simulink model "case3"  (R2024b)
settings: Solver=FixedStepAuto  StartTime=0  StopTime=1  FixedStep=1e-7  RelTol=1e-3
values from neighbouring files (symbols this model uses):
  SG_D_1_D = 0.01056    [IEEE9_case_parameters.m]    (also in case1_parameters.m; case2_parameters.m; case3_parameters.m; case4_parameters.m)
  SG_D_1_EnableSaturation = 0    [IEEE9_case_parameters.m]    (also in case1_parameters.m; case2_parameters.m; case3_parameters.m; case4_parameters.m)
  SG_D_1_f0 = 60    [IEEE9_case_parameters.m]    (also in case1_parameters.m; case2_parameters.m; case3_parameters.m; case4_parameters.m)
  SG_D_1_H = 7.5    [IEEE9_case_parameters.m]    (also in case1_parameters.m; case2_parameters.m; case3_parameters.m; case4_parameters.m)
  SG_D_1_K_A = 20    [IEEE9_case_parameters.m]    (also in case1_parameters.m; case2_parameters.m; case3_parameters.m; case4_parameters.m)
  SG_D_1_K_E = 1.000000e+1    (= 10)    [IEEE9_case_parameters.m]    (also in case1_parameters.m; case2_parameters.m; case3_parameters.m; case4_parameters.m)
  SG_D_1_K_F = 2.363    [IEEE9_case_parameters.m]    (also in case1_parameters.m; case2_parameters.m; case3_parameters.m; case4_parameters.m)
  SG_D_1_K_s = 0.5    [IEEE9_case_parameters.m]    (also in case1_parameters.m = 5; case2_parameters.m = 5; case3_parameters.m = 5; case4_parameters.m = 5)
  SG_D_1_R_a = 0.001088    [IEEE9_case_parameters.m]    (also in case1_parameters.m; case2_parameters.m; case3_parameters.m; case4_parameters.m)
  SG_D_1_S_A = 1    [IEEE9_case_parameters.m]    (also in case1_parameters.m; case2_parameters.m; case3_parameters.m; case4_parameters.m)
  SG_D_1_S_B = 0.103    [IEEE9_case_parameters.m]    (also in case1_parameters.m; case2_parameters.m; case3_parameters.m; case4_parameters.m)
  SG_D_1_S_N = 10.659857    [IEEE9_case_parameters.m]    (also in case1_parameters.m; case2_parameters.m; case3_parameters.m; case4_parameters.m)
  SG_D_1_SpeedPara = 200    [IEEE9_case_parameters.m]    (also in case1_parameters.m; case2_parameters.m; case3_parameters.m; case4_parameters.m)
  SG_D_1_T_0 = 0.720173    [IEEE9_case_parameters.m]    (also in case1_parameters.m = 0.755522; case2_parameters.m = 0.808931; case3_parameters.m = 0.869402; case4_parameters.m = 0.729316)
  SG_D_1_T_1 = 0.3    [IEEE9_case_parameters.m]    (also in case1_parameters.m; case2_parameters.m; case3_parameters.m; case4_parameters.m)
  SG_D_1_T_2 = 0.05    [IEEE9_case_parameters.m]    (also in case1_parameters.m; case2_parameters.m; case3_parameters.m; case4_parameters.m)
  SG_D_1_T_3 = 0.02    [IEEE9_case_parameters.m]    (also in case1_parameters.m; case2_parameters.m; case3_parameters.m; case4_parameters.m)
  SG_D_1_T_4 = 0.005    [IEEE9_case_parameters.m]    (also in case1_parameters.m; case2_parameters.m; case3_parameters.m; case4_parameters.m)
  SG_D_1_T_A = 0.02    [IEEE9_case_parameters.m]    (also in case1_parameters.m; case2_parameters.m; case3_parameters.m; case4_parameters.m)
  SG_D_1_T_dd = 8.000000e+0    (= 8)    [IEEE9_case_parameters.m]    (also in case1_parameters.m; case2_parameters.m; case3_parameters.m; case4_parameters.m)
  SG_D_1_T_ddd = 0.04    [IEEE9_case_parameters.m]    (also in case1_parameters.m; case2_parameters.m; case3_parameters.m; case4_parameters.m)
  SG_D_1_T_E = 0.314    [IEEE9_case_parameters.m]    (also in case1_parameters.m; case2_parameters.m; case3_parameters.m; case4_parameters.m)
  SG_D_1_T_F = 0.35    [IEEE9_case_parameters.m]    (also in case1_parameters.m; case2_parameters.m; case3_parameters.m; case4_parameters.m)
  SG_D_1_T_qd = 0.8    [IEEE9_case_parameters.m]    (also in case1_parameters.m; case2_parameters.m; case3_parameters.m; case4_parameters.m)
  SG_D_1_T_qdd = 0.02    [IEEE9_case_parameters.m]    (also in case1_parameters.m; case2_parameters.m; case3_parameters.m; case4_parameters.m)
  SG_D_1_T_speed = 0.1    [IEEE9_case_parameters.m]    (also in case1_parameters.m = 200; case2_parameters.m = 200; case3_parameters.m = 200; case4_parameters.m = 200)
  SG_D_1_T_w = 0.5    [IEEE9_case_parameters.m]    (also in case1_parameters.m; case2_parameters.m; case3_parameters.m; case4_parameters.m)
  SG_D_1_V_ref = 1.990276    [IEEE9_case_parameters.m]    (also in case1_parameters.m = 2.042296; case2_parameters.m = 2.051388; case3_parameters.m = 2.089584; case4_parameters.m = 2.01845)
  SG_D_1_w_ref = 376.991118    [IEEE9_case_parameters.m]    (also in case1_parameters.m; case2_parameters.m; case3_parameters.m; case4_parameters.m)
  SG_D_1_wb = 6.000000e+1    (= 60)    [IEEE9_case_parameters.m]    (also in case1_parameters.m; case2_parameters.m; case3_parameters.m; case4_parameters.m)
  SG_D_1_x_d = 1.9    [IEEE9_case_parameters.m]    (also in case1_parameters.m; case2_parameters.m; case3_parameters.m; case4_parameters.m)
  SG_D_1_x_dd = 0.302    [IEEE9_case_parameters.m]    (also in case1_parameters.m; case2_parameters.m; case3_parameters.m; case4_parameters.m)
  SG_D_1_x_ddd = 0.204    [IEEE9_case_parameters.m]    (also in case1_parameters.m; case2_parameters.m; case3_parameters.m; case4_parameters.m)
  SG_D_1_x_l = 0.05    [IEEE9_case_parameters.m]    (also in case1_parameters.m; case2_parameters.m; case3_parameters.m; case4_parameters.m)
  SG_D_1_x_q = 1.3    [IEEE9_case_parameters.m]    (also in case1_parameters.m; case2_parameters.m; case3_parameters.m; case4_parameters.m)
  SG_D_1_x_qd = 0.5    [IEEE9_case_parameters.m]    (also in case1_parameters.m; case2_parameters.m; case3_parameters.m; case4_parameters.m)
  SG_D_1_x_qdd = 0.3    [IEEE9_case_parameters.m]    (also in case1_parameters.m; case2_parameters.m; case3_parameters.m; case4_parameters.m)
  SG_D_2_D = 0.02    [IEEE9_case_parameters.m]    (also in case1_parameters.m; case2_parameters.m; case3_parameters.m; case4_parameters.m)
  SG_D_2_EnableSaturation = 0    [IEEE9_case_parameters.m]    (also in case1_parameters.m; case2_parameters.m; case3_parameters.m; case4_parameters.m)
  SG_D_2_f0 = 60    [IEEE9_case_parameters.m]    (also in case1_parameters.m; case2_parameters.m; case3_parameters.m; case4_parameters.m)
  SG_D_2_H = 8.000000e+0    (= 8)    [IEEE9_case_parameters.m]    (also in case1_parameters.m; case2_parameters.m; case3_parameters.m; case4_parameters.m)
  SG_D_2_K_A = 20    [IEEE9_case_parameters.m]    (also in case1_parameters.m; case2_parameters.m; case3_parameters.m; case4_parameters.m)
  SG_D_2_K_E = 1.000000e+1    (= 10)    [IEEE9_case_parameters.m]    (also in case1_parameters.m; case2_parameters.m; case3_parameters.m; case4_parameters.m)
  SG_D_2_K_F = 2.363    [IEEE9_case_parameters.m]    (also in case1_parameters.m; case2_parameters.m; case3_parameters.m; case4_parameters.m)
  SG_D_2_K_s = 0.5    [IEEE9_case_parameters.m]    (also in case1_parameters.m = 4; case2_parameters.m = 4; case3_parameters.m = 4; case4_parameters.m = 4)
  SG_D_2_R_a = 0.001088    [IEEE9_case_parameters.m]    (also in case1_parameters.m; case2_parameters.m; case3_parameters.m; case4_parameters.m)
  SG_D_2_S_A = 1    [IEEE9_case_parameters.m]    (also in case1_parameters.m; case2_parameters.m; case3_parameters.m; case4_parameters.m)
  SG_D_2_S_B = 0.103    [IEEE9_case_parameters.m]    (also in case1_parameters.m; case2_parameters.m; case3_parameters.m; case4_parameters.m)
  SG_D_2_S_N = 10.659857    [IEEE9_case_parameters.m]    (also in case1_parameters.m; case2_parameters.m; case3_parameters.m; case4_parameters.m)
  SG_D_2_SpeedPara = 200    [IEEE9_case_parameters.m]    (also in case1_parameters.m; case2_parameters.m; case3_parameters.m; case4_parameters.m)
  SG_D_2_T_0 = 1.632913    [IEEE9_case_parameters.m]    (also in case1_parameters.m = 1.632925; case2_parameters.m = 1.632915; case3_parameters.m = 1.632914; case4_parameters.m = 1.632927)
  SG_D_2_T_1 = 0.2    [IEEE9_case_parameters.m]    (also in case1_parameters.m; case2_parameters.m; case3_parameters.m; case4_parameters.m)
  SG_D_2_T_2 = 0.05    [IEEE9_case_parameters.m]    (also in case1_parameters.m; case2_parameters.m; case3_parameters.m; case4_parameters.m)
  SG_D_2_T_3 = 0.02    [IEEE9_case_parameters.m]    (also in case1_parameters.m; case2_parameters.m; case3_parameters.m; case4_parameters.m)
  SG_D_2_T_4 = 0.005    [IEEE9_case_parameters.m]    (also in case1_parameters.m; case2_parameters.m; case3_parameters.m; case4_parameters.m)
  SG_D_2_T_A = 0.02    [IEEE9_case_parameters.m]    (also in case1_parameters.m; case2_parameters.m; case3_parameters.m; case4_parameters.m)
  SG_D_2_T_dd = 7.9    [IEEE9_case_parameters.m]    (also in case1_parameters.m; case2_parameters.m; case3_parameters.m; case4_parameters.m)
  SG_D_2_T_ddd = 0.04    [IEEE9_case_parameters.m]    (also in case1_parameters.m; case2_parameters.m; case3_parameters.m; case4_parameters.m)
  SG_D_2_T_E = 0.314    [IEEE9_case_parameters.m]    (also in case1_parameters.m; case2_parameters.m; case3_parameters.m; case4_parameters.m)
  SG_D_2_T_F = 0.35    [IEEE9_case_parameters.m]    (also in case1_parameters.m; case2_parameters.m; case3_parameters.m; case4_parameters.m)
  SG_D_2_T_qd = 0.8    [IEEE9_case_parameters.m]    (also in case1_parameters.m; case2_parameters.m; case3_parameters.m; case4_parameters.m)
  SG_D_2_T_qdd = 0.015    [IEEE9_case_parameters.m]    (also in case1_parameters.m; case2_parameters.m; case3_parameters.m; case4_parameters.m)
  SG_D_2_T_speed = 0.1    [IEEE9_case_parameters.m]    (also in case1_parameters.m = 150; case2_parameters.m = 150; case3_parameters.m = 150; case4_parameters.m = 150)
  SG_D_2_T_w = 0.35    [IEEE9_case_parameters.m]    (also in case1_parameters.m; case2_parameters.m; case3_parameters.m; case4_parameters.m)
  SG_D_2_V_ref = 2.58547    [IEEE9_case_parameters.m]    (also in case1_parameters.m = 2.597896; case2_parameters.m = 2.587136; case3_parameters.m = 2.586042; case4_parameters.m = 2.599679)
  SG_D_2_w_ref = 376.991118    [IEEE9_case_parameters.m]    (also in case1_parameters.m; case2_parameters.m; case3_parameters.m; case4_parameters.m)
  SG_D_2_wb = 6.000000e+1    (= 60)    [IEEE9_case_parameters.m]    (also in case1_parameters.m; case2_parameters.m; case3_parameters.m; case4_parameters.m)
  SG_D_2_x_d = 1.8    [IEEE9_case_parameters.m]    (also in case1_parameters.m; case2_parameters.m; case3_parameters.m; case4_parameters.m)
  SG_D_2_x_dd = 0.302    [IEEE9_case_parameters.m]    (also in case1_parameters.m; case2_parameters.m; case3_parameters.m; case4_parameters.m)
  SG_D_2_x_ddd = 0.204    [IEEE9_case_parameters.m]    (also in case1_parameters.m; case2_parameters.m; case3_parameters.m; case4_parameters.m)
  SG_D_2_x_l = 0.05    [IEEE9_case_parameters.m]    (also in case1_parameters.m; case2_parameters.m; case3_parameters.m; case4_parameters.m)
  SG_D_2_x_q = 1.25    [IEEE9_case_parameters.m]    (also in case1_parameters.m; case2_parameters.m; case3_parameters.m; case4_parameters.m)
  SG_D_2_x_qd = 0.5    [IEEE9_case_parameters.m]    (also in case1_parameters.m; case2_parameters.m; case3_parameters.m; case4_parameters.m)
  SG_D_2_x_qdd = 0.3    [IEEE9_case_parameters.m]    (also in case1_parameters.m; case2_parameters.m; case3_parameters.m; case4_parameters.m)
  SG_D_3_D = 0.02    [IEEE9_case_parameters.m]    (also in case1_parameters.m; case2_parameters.m; case3_parameters.m; case4_parameters.m)
  SG_D_3_EnableSaturation = 0    [IEEE9_case_parameters.m]    (also in case1_parameters.m; case2_parameters.m; case3_parameters.m; case4_parameters.m)
  SG_D_3_f0 = 60    [IEEE9_case_parameters.m]    (also in case1_parameters.m; case2_parameters.m; case3_parameters.m; case4_parameters.m)
  SG_D_3_H = 7.7    [IEEE9_case_parameters.m]    (also in case1_parameters.m; case2_parameters.m; case3_parameters.m; case4_parameters.m)
  SG_D_3_K_A = 20    [IEEE9_case_parameters.m]    (also in case1_parameters.m; case2_parameters.m; case3_parameters.m; case4_parameters.m)
  SG_D_3_K_E = 1.000000e+1    (= 10)    [IEEE9_case_parameters.m]    (also in case1_parameters.m; case2_parameters.m; case3_parameters.m; case4_parameters.m)
  SG_D_3_K_F = 2.363    [IEEE9_case_parameters.m]    (also in case1_parameters.m; case2_parameters.m; case3_parameters.m; case4_parameters.m)
  SG_D_3_K_s = 0.2    [IEEE9_case_parameters.m]    (also in case1_parameters.m = 2; case2_parameters.m = 2; case3_parameters.m = 2; case4_parameters.m = 2)
  SG_D_3_R_a = 0.001088    [IEEE9_case_parameters.m]    (also in case1_parameters.m; case2_parameters.m; case3_parameters.m; case4_parameters.m)
  SG_D_3_S_A = 1    [IEEE9_case_parameters.m]    (also in case1_parameters.m; case2_parameters.m; case3_parameters.m; case4_parameters.m)
  SG_D_3_S_B = 0.103    [IEEE9_case_parameters.m]    (also in case1_parameters.m; case2_parameters.m; case3_parameters.m; case4_parameters.m)
  SG_D_3_S_N = 10.659857    [IEEE9_case_parameters.m]    (also in case1_parameters.m; case2_parameters.m; case3_parameters.m; case4_parameters.m)
  SG_D_3_SpeedPara = 200    [IEEE9_case_parameters.m]    (also in case1_parameters.m; case2_parameters.m; case3_parameters.m; case4_parameters.m)
  SG_D_3_T_0 = 0.850788    [IEEE9_case_parameters.m]    (also in case1_parameters.m = 0.850786; case2_parameters.m = 0.850787; case3_parameters.m; case4_parameters.m = 0.850786)
  SG_D_3_T_1 = 0.2    [IEEE9_case_parameters.m]    (also in case1_parameters.m; case2_parameters.m; case3_parameters.m; case4_parameters.m)
  SG_D_3_T_2 = 0.05    [IEEE9_case_parameters.m]    (also in case1_parameters.m; case2_parameters.m; case3_parameters.m; case4_parameters.m)
  SG_D_3_T_3 = 0.02    [IEEE9_case_parameters.m]    (also in case1_parameters.m; case2_parameters.m; case3_parameters.m; case4_parameters.m)
  SG_D_3_T_4 = 0.005    [IEEE9_case_parameters.m]    (also in case1_parameters.m; case2_parameters.m; case3_parameters.m; case4_parameters.m)
  SG_D_3_T_A = 0.02    [IEEE9_case_parameters.m]    (also in case1_parameters.m; case2_parameters.m; case3_parameters.m; case4_parameters.m)
  SG_D_3_T_dd = 8.1    [IEEE9_case_parameters.m]    (also in case1_parameters.m; case2_parameters.m; case3_parameters.m; case4_parameters.m)
  SG_D_3_T_ddd = 0.04    [IEEE9_case_parameters.m]    (also in case1_parameters.m; case2_parameters.m; case3_parameters.m; case4_parameters.m)
  SG_D_3_T_E = 0.314    [IEEE9_case_parameters.m]    (also in case1_parameters.m; case2_parameters.m; case3_parameters.m; case4_parameters.m)
  SG_D_3_T_F = 0.35    [IEEE9_case_parameters.m]    (also in case1_parameters.m; case2_parameters.m; case3_parameters.m; case4_parameters.m)
  SG_D_3_T_qd = 0.8    [IEEE9_case_parameters.m]    (also in case1_parameters.m; case2_parameters.m; case3_parameters.m; case4_parameters.m)
  SG_D_3_T_qdd = 0.015    [IEEE9_case_parameters.m]    (also in case1_parameters.m; case2_parameters.m; case3_parameters.m; case4_parameters.m)
  SG_D_3_T_speed = 0.1    [IEEE9_case_parameters.m]    (also in case1_parameters.m = 180; case2_parameters.m = 180; case3_parameters.m = 180; case4_parameters.m = 180)
  SG_D_3_T_w = 0.4    [IEEE9_case_parameters.m]    (also in case1_parameters.m; case2_parameters.m; case3_parameters.m; case4_parameters.m)
  SG_D_3_V_ref = 1.892727    [IEEE9_case_parameters.m]    (also in case1_parameters.m = 1.906439; case2_parameters.m = 1.895535; case3_parameters.m = 1.892105; case4_parameters.m = 1.906598)
  SG_D_3_w_ref = 376.991118    [IEEE9_case_parameters.m]    (also in case1_parameters.m; case2_parameters.m; case3_parameters.m; case4_parameters.m)
  SG_D_3_wb = 6.000000e+1    (= 60)    [IEEE9_case_parameters.m]    (also in case1_parameters.m; case2_parameters.m; case3_parameters.m; case4_parameters.m)
  SG_D_3_x_d = 1.85    [IEEE9_case_parameters.m]    (also in case1_parameters.m; case2_parameters.m; case3_parameters.m; case4_parameters.m)
  SG_D_3_x_dd = 0.302    [IEEE9_case_parameters.m]    (also in case1_parameters.m; case2_parameters.m; case3_parameters.m; case4_parameters.m)
  SG_D_3_x_ddd = 0.204    [IEEE9_case_parameters.m]    (also in case1_parameters.m; case2_parameters.m; case3_parameters.m; case4_parameters.m)
  SG_D_3_x_l = 0.05    [IEEE9_case_parameters.m]    (also in case1_parameters.m; case2_parameters.m; case3_parameters.m; case4_parameters.m)
  SG_D_3_x_q = 1.2    [IEEE9_case_parameters.m]    (also in case1_parameters.m; case2_parameters.m; case3_parameters.m; case4_parameters.m)
  SG_D_3_x_qd = 0.5    [IEEE9_case_parameters.m]    (also in case1_parameters.m; case2_parameters.m; case3_parameters.m; case4_parameters.m)
  SG_D_3_x_qdd = 0.3    [IEEE9_case_parameters.m]    (also in case1_parameters.m; case2_parameters.m; case3_parameters.m; case4_parameters.m)
(part 2 of 12)

== system case3/SG_D_2 ==
  v_d_SG_D_2 : Inport
  v_q_SG_D_2 : Inport  Port=2
  E_fd_SG_D_2 : Integrator  InitialCondition=3.1720837123564576
  Px_1_SG_D_2 : Integrator  InitialCondition=0.0
  Px_2_SG_D_2 : Integrator  InitialCondition=0.0
  Px_3_SG_D_2 : Integrator  InitialCondition=-5.706943293029926e-25
  R_f_SG_D_2 : Integrator  InitialCondition=21.416096606566597
  T_e_SG_D_2_block : Subsystem
  T_m_SG_D_2 : Integrator  InitialCondition=1.6329139534534778
  V_f_SG_D_2 : Integrator  InitialCondition=31.720837123564575
  d_E_fd_SG_D_2_block : Subsystem
  d_Px_1_SG_D_2_block : Subsystem
  d_Px_2_SG_D_2_block : Subsystem
  d_Px_3_SG_D_2_block : Subsystem
  d_R_f_SG_D_2_block : Subsystem
  d_T_m_SG_D_2_block : Subsystem
  d_V_f_SG_D_2_block : Subsystem
  d_psi_1d_SG_D_2_block : Subsystem
  d_psi_d_SG_D_2_block : Subsystem
  d_psi_fd_SG_D_2_block : Subsystem
  d_psi_gq_SG_D_2_block : Subsystem
  d_psi_kq_SG_D_2_block : Subsystem
  d_psi_q_SG_D_2_block : Subsystem
  d_theta_SG_D_2_block : Subsystem
  d_w_SG_D_2_block : Subsystem
  i_d_SG_D_2_block : Subsystem
  i_q_SG_D_2_block : Subsystem
  psi_1d_SG_D_2 : Integrator  InitialCondition=0.577501053237212
  psi_d_SG_D_2 : Integrator  InitialCondition=0.5033701201195192
  psi_fd_SG_D_2 : Integrator  InitialCondition=0.9511209561503834
  psi_gq_SG_D_2 : Integrator  InitialCondition=0.5196736341788188
  psi_kq_SG_D_2 : Integrator  InitialCondition=-0.8314778146861102
  psi_q_SG_D_2 : Integrator  InitialCondition=-0.8661227236313648
  theta_SG_D_2 : Integrator  InitialCondition=1.1998359576141482
  theta_SG_D_2_out_block : Subsystem
  w_SG_D_2 : Integrator  InitialCondition=376.99111843077515
  w_SG_D_2_out_block : Subsystem
  i_d_SG_D_2 : Outport
  i_q_SG_D_2 : Outport  Port=2
  T_e_SG_D_2 : Outport  Port=3
  w_SG_D_2_out : Outport  Port=4
  theta_SG_D_2_out : Outport  Port=5
  wires:
  T_e_SG_D_2_block/1(Blockout_T_e_SG_D_2_f9887) -> T_e_SG_D_2/1
  d_Px_2_SG_D_2_block/1(Blockout_d_Px_2_SG_D_2_1ade1) -> Px_2_SG_D_2/1
  d_T_m_SG_D_2_block/1(Blockout_d_T_m_SG_D_2_41985) -> T_m_SG_D_2/1
  w_SG_D_2/1 -> d_psi_q_SG_D_2_block/9(State_w_SG_D_2_01d6c), d_w_SG_D_2_block/1(State_w_SG_D_2_02aad), d_V_f_SG_D_2_block/8(State_w_SG_D_2_f63e0), d_psi_d_SG_D_2_block/9(State_w_SG_D_2_5f49e), d_V_f_SG_D_2_block/13(State_w_SG_D_2_1a1a5), d_T_m_SG_D_2_block/1(State_w_SG_D_2_a6fad), d_theta_SG_D_2_block/1(State_w_SG_D_2_906f7), d_Px_2_SG_D_2_block/4(State_w_SG_D_2_0d46f), d_Px_1_SG_D_2_block/2(State_w_SG_D_2_bbb39), d_Px_3_SG_D_2_block/6(State_w_SG_D_2_22dc6), w_SG_D_2_out_block/1(State_w_SG_D_2_ed650)
  d_Px_3_SG_D_2_block/1(Blockout_d_Px_3_SG_D_2_2b25a) -> Px_3_SG_D_2/1
  d_Px_1_SG_D_2_block/1(Blockout_d_Px_1_SG_D_2_109b7) -> Px_1_SG_D_2/1
  d_theta_SG_D_2_block/1(Blockout_d_theta_SG_D_2_79f4e) -> theta_SG_D_2/1
  psi_q_SG_D_2/1 -> d_psi_d_SG_D_2_block/8(State_psi_q_SG_D_2_f5763), d_psi_q_SG_D_2_block/3(State_psi_q_SG_D_2_7ccdb), d_psi_gq_SG_D_2_block/9(State_psi_q_SG_D_2_77370), d_psi_kq_SG_D_2_block/5(State_psi_q_SG_D_2_baf03), d_V_f_SG_D_2_block/11(State_psi_q_SG_D_2_26ca5), d_V_f_SG_D_2_block/7(State_psi_q_SG_D_2_6efa9), d_w_SG_D_2_block/7(State_psi_q_SG_D_2_2b35c), d_psi_gq_SG_D_2_block/6(State_psi_q_SG_D_2_cf3b4), d_w_SG_D_2_block/6(State_psi_q_SG_D_2_f2b6f), i_d_SG_D_2_block/3(State_psi_q_SG_D_2_858f7), i_q_SG_D_2_block/3(State_psi_q_SG_D_2_1cc4f), T_e_SG_D_2_block/4(State_psi_q_SG_D_2_fc5b5), T_e_SG_D_2_block/5(State_psi_q_SG_D_2_0409e)
  w_SG_D_2_out_block/1(Blockout_w_SG_D_2_out_9b37d) -> w_SG_D_2_out/1
  psi_gq_SG_D_2/1 -> d_psi_q_SG_D_2_block/1(State_psi_gq_SG_D_2_0e848), d_psi_gq_SG_D_2_block/2(State_psi_gq_SG_D_2_6a3ed), d_psi_kq_SG_D_2_block/1(State_psi_gq_SG_D_2_f7272), d_w_SG_D_2_block/4(State_psi_gq_SG_D_2_e9134), d_V_f_SG_D_2_block/9(State_psi_gq_SG_D_2_b760b), i_q_SG_D_2_block/1(State_psi_gq_SG_D_2_7b19c), i_d_SG_D_2_block/1(State_psi_gq_SG_D_2_2ee45), d_psi_gq_SG_D_2_block/4(State_psi_gq_SG_D_2_31acd), d_psi_kq_SG_D_2_block/3(State_psi_gq_SG_D_2_fd868), d_psi_gq_SG_D_2_block/1(State_psi_gq_SG_D_2_6e475), T_e_SG_D_2_block/2(State_psi_gq_SG_D_2_7cf1b), d_psi_gq_SG_D_2_block/7(State_psi_gq_SG_D_2_de864)
  psi_1d_SG_D_2/1 -> d_psi_fd_SG_D_2_block/3(State_psi_1d_SG_D_2_7e7b9), d_psi_fd_SG_D_2_block/8(State_psi_1d_SG_D_2_9ae7e), d_psi_fd_SG_D_2_block/5(State_psi_1d_SG_D_2_899e2), d_psi_d_SG_D_2_block/1(State_psi_1d_SG_D_2_d85f5), d_psi_1d_SG_D_2_block/3(State_psi_1d_SG_D_2_3fe79), i_d_SG_D_2_block/5(State_psi_1d_SG_D_2_56a6d), i_q_SG_D_2_block/5(State_psi_1d_SG_D_2_4f110), d_V_f_SG_D_2_block/4(State_psi_1d_SG_D_2_c35c0), d_psi_1d_SG_D_2_block/1(State_psi_1d_SG_D_2_b7293), T_e_SG_D_2_block/6(State_psi_1d_SG_D_2_3067b), d_w_SG_D_2_block/8(State_psi_1d_SG_D_2_8e36d)
  T_m_SG_D_2/1 -> d_T_m_SG_D_2_block/2(State_T_m_SG_D_2_ffd37), d_w_SG_D_2_block/2(State_T_m_SG_D_2_487f3)
  Px_2_SG_D_2/1 -> d_Px_3_SG_D_2_block/2(State_Px_2_SG_D_2_c1187), d_Px_2_SG_D_2_block/1(State_Px_2_SG_D_2_a9fab), d_Px_3_SG_D_2_block/3(State_Px_2_SG_D_2_e6f9b)
  v_d_SG_D_2/1 -> d_psi_d_SG_D_2_block/4(Input_v_d_SG_D_2_8a747), d_psi_q_SG_D_2_block/4(Input_v_d_SG_D_2_cf2d7)
  theta_SG_D_2/1 -> d_psi_q_SG_D_2_block/5(State_theta_SG_D_2_ef5e0), i_d_SG_D_2_block/8(State_theta_SG_D_2_96e4e), d_psi_d_SG_D_2_block/5(State_theta_SG_D_2_fc879), i_q_SG_D_2_block/4(State_theta_SG_D_2_75646), i_d_SG_D_2_block/4(State_theta_SG_D_2_26ddd), i_q_SG_D_2_block/8(State_theta_SG_D_2_3ab4c), d_psi_d_SG_D_2_block/7(State_theta_SG_D_2_1886b), theta_SG_D_2_out_block/1(State_theta_SG_D_2_c18fe), d_psi_q_SG_D_2_block/7(State_theta_SG_D_2_f1f7c)
  d_V_f_SG_D_2_block/1(Blockout_d_V_f_SG_D_2_ae7dd) -> V_f_SG_D_2/1
  v_q_SG_D_2/1 -> d_psi_d_SG_D_2_block/6(Input_v_q_SG_D_2_bd396), d_psi_q_SG_D_2_block/6(Input_v_q_SG_D_2_6f15e)
  Px_1_SG_D_2/1 -> d_Px_1_SG_D_2_block/1(State_Px_1_SG_D_2_e1673), d_Px_3_SG_D_2_block/4(State_Px_1_SG_D_2_d9778), d_Px_2_SG_D_2_block/3(State_Px_1_SG_D_2_ca2a4), d_Px_2_SG_D_2_block/2(State_Px_1_SG_D_2_b7eac), d_Px_3_SG_D_2_block/5(State_Px_1_SG_D_2_e27f8)
  i_d_SG_D_2_block/1(Blockout_i_d_SG_D_2_b1c5f) -> i_d_SG_D_2/1
  psi_d_SG_D_2/1 -> d_psi_fd_SG_D_2_block/6(State_psi_d_SG_D_2_990fd), d_psi_fd_SG_D_2_block/9(State_psi_d_SG_D_2_3b4a4), d_psi_q_SG_D_2_block/8(State_psi_d_SG_D_2_a8ebf), d_psi_1d_SG_D_2_block/4(State_psi_d_SG_D_2_4a3d7), d_V_f_SG_D_2_block/5(State_psi_d_SG_D_2_fa29d), d_V_f_SG_D_2_block/12(State_psi_d_SG_D_2_5cd6e), d_w_SG_D_2_block/3(State_psi_d_SG_D_2_ff7e2), i_d_SG_D_2_block/6(State_psi_d_SG_D_2_e3a72), T_e_SG_D_2_block/1(State_psi_d_SG_D_2_bd8f2), T_e_SG_D_2_block/7(State_psi_d_SG_D_2_0f14f), d_psi_d_SG_D_2_block/2(State_psi_d_SG_D_2_2712a), i_q_SG_D_2_block/6(State_psi_d_SG_D_2_a879f), d_w_SG_D_2_block/9(State_psi_d_SG_D_2_34d9a)
  psi_kq_SG_D_2/1 -> d_psi_gq_SG_D_2_block/3(State_psi_kq_SG_D_2_65b80), d_psi_q_SG_D_2_block/2(State_psi_kq_SG_D_2_c82e0), d_psi_gq_SG_D_2_block/5(State_psi_kq_SG_D_2_4f33d), d_psi_kq_SG_D_2_block/2(State_psi_kq_SG_D_2_8e84a), d_psi_kq_SG_D_2_block/4(State_psi_kq_SG_D_2_a3af5), d_psi_gq_SG_D_2_block/8(State_psi_kq_SG_D_2_af7b7), d_w_SG_D_2_block/5(State_psi_kq_SG_D_2_55a18), i_d_SG_D_2_block/2(State_psi_kq_SG_D_2_8f947), i_q_SG_D_2_block/2(State_psi_kq_SG_D_2_0c2bc), d_V_f_SG_D_2_block/10(State_psi_kq_SG_D_2_27cac), T_e_SG_D_2_block/3(State_psi_kq_SG_D_2_00a62)
  psi_fd_SG_D_2/1 -> d_psi_fd_SG_D_2_block/7(State_psi_fd_SG_D_2_f0ae5), d_psi_fd_SG_D_2_block/10(State_psi_fd_SG_D_2_a82ed), d_psi_fd_SG_D_2_block/4(State_psi_fd_SG_D_2_eba15), d_psi_d_SG_D_2_block/3(State_psi_fd_SG_D_2_3f7c9), d_psi_1d_SG_D_2_block/5(State_psi_fd_SG_D_2_5dfd6), d_psi_fd_SG_D_2_block/2(State_psi_fd_SG_D_2_f7b95), i_d_SG_D_2_block/7(State_psi_fd_SG_D_2_d0a13), d_V_f_SG_D_2_block/6(State_psi_fd_SG_D_2_17c38), i_q_SG_D_2_block/7(State_psi_fd_SG_D_2_1b685), d_w_SG_D_2_block/10(State_psi_fd_SG_D_2_06bb8), d_psi_1d_SG_D_2_block/2(State_psi_fd_SG_D_2_8ed55), T_e_SG_D_2_block/8(State_psi_fd_SG_D_2_e1184)
  d_R_f_SG_D_2_block/1(Blockout_d_R_f_SG_D_2_d9bc5) -> R_f_SG_D_2/1
  d_w_SG_D_2_block/1(Blockout_d_w_SG_D_2_8967f) -> w_SG_D_2/1
  R_f_SG_D_2/1 -> d_V_f_SG_D_2_block/2(State_R_f_SG_D_2_ef74e), d_R_f_SG_D_2_block/2(State_R_f_SG_D_2_45923)
  theta_SG_D_2_out_block/1(Blockout_theta_SG_D_2_out_3c0c9) -> theta_SG_D_2_out/1
  d_psi_q_SG_D_2_block/1(Blockout_d_psi_q_SG_D_2_96569) -> psi_q_SG_D_2/1
  d_psi_d_SG_D_2_block/1(Blockout_d_psi_d_SG_D_2_7b72e) -> psi_d_SG_D_2/1
  i_q_SG_D_2_block/1(Blockout_i_q_SG_D_2_91d2d) -> i_q_SG_D_2/1
  d_psi_1d_SG_D_2_block/1(Blockout_d_psi_1d_SG_D_2_dad19) -> psi_1d_SG_D_2/1
  d_psi_gq_SG_D_2_block/1(Blockout_d_psi_gq_SG_D_2_d0f45) -> psi_gq_SG_D_2/1
  d_psi_kq_SG_D_2_block/1(Blockout_d_psi_kq_SG_D_2_93807) -> psi_kq_SG_D_2/1
  V_f_SG_D_2/1 -> d_V_f_SG_D_2_block/14(State_V_f_SG_D_2_a9119), d_E_fd_SG_D_2_block/2(State_V_f_SG_D_2_75a88)
  Px_3_SG_D_2/1 -> d_Px_3_SG_D_2_block/1(State_Px_3_SG_D_2_127e3), d_V_f_SG_D_2_block/3(State_Px_3_SG_D_2_c6752)
  d_E_fd_SG_D_2_block/1(Blockout_d_E_fd_SG_D_2_c4f8a) -> E_fd_SG_D_2/1
  E_fd_SG_D_2/1 -> d_V_f_SG_D_2_block/1(State_E_fd_SG_D_2_ed342), d_E_fd_SG_D_2_block/1(State_E_fd_SG_D_2_aeb78), d_psi_fd_SG_D_2_block/1(State_E_fd_SG_D_2_53335), d_R_f_SG_D_2_block/1(State_E_fd_SG_D_2_79ff1)
  d_psi_fd_SG_D_2_block/1(Blockout_d_psi_fd_SG_D_2_efff3) -> psi_fd_SG_D_2/1

== system case3/SG_D_3 ==
  v_d_SG_D_3 : Inport
  v_q_SG_D_3 : Inport  Port=2
  E_fd_SG_D_3 : Integrator  InitialCondition=1.7842098420554462
  Px_1_SG_D_3 : Integrator  InitialCondition=0.0
  Px_2_SG_D_3 : Integrator  InitialCondition=0.0
  Px_3_SG_D_3 : Integrator  InitialCondition=-4.774407798544695e-24
  R_f_SG_D_3 : Integrator  InitialCondition=12.045965305077198
  T_e_SG_D_3_block : Subsystem
  T_m_SG_D_3 : Integrator  InitialCondition=0.8507876281015136
  V_f_SG_D_3 : Integrator  InitialCondition=17.84209842055446
  d_E_fd_SG_D_3_block : Subsystem
  d_Px_1_SG_D_3_block : Subsystem
  d_Px_2_SG_D_3_block : Subsystem
  d_Px_3_SG_D_3_block : Subsystem
  d_R_f_SG_D_3_block : Subsystem
  d_T_m_SG_D_3_block : Subsystem
  d_V_f_SG_D_3_block : Subsystem
  d_psi_1d_SG_D_3_block : Subsystem
  d_psi_d_SG_D_3_block : Subsystem
  d_psi_fd_SG_D_3_block : Subsystem
  d_psi_gq_SG_D_3_block : Subsystem
  d_psi_kq_SG_D_3_block : Subsystem
  d_psi_q_SG_D_3_block : Subsystem
  d_theta_SG_D_3_block : Subsystem
  d_w_SG_D_3_block : Subsystem
  i_d_SG_D_3_block : Subsystem
  i_q_SG_D_3_block : Subsystem
  psi_1d_SG_D_3 : Integrator  InitialCondition=0.7140925496692515
  psi_d_SG_D_3 : Integrator  InitialCondition=0.6843670693251905
  psi_fd_SG_D_3 : Integrator  InitialCondition=0.8639089706033187
  psi_gq_SG_D_3 : Integrator  InitialCondition=0.42606986581987333
  psi_kq_SG_D_3 : Integrator  InitialCondition=-0.6999719224183634
  psi_q_SG_D_3 : Integrator  InitialCondition=-0.73040548426264
  theta_SG_D_3 : Integrator  InitialCondition=0.8848466613207072
  theta_SG_D_3_out_block : Subsystem
  w_SG_D_3 : Integrator  InitialCondition=376.99111843077515
  w_SG_D_3_out_block : Subsystem
  i_d_SG_D_3 : Outport
  i_q_SG_D_3 : Outport  Port=2
  T_e_SG_D_3 : Outport  Port=3
  w_SG_D_3_out : Outport  Port=4
  theta_SG_D_3_out : Outport  Port=5
  wires:
  d_Px_1_SG_D_3_block/1(Blockout_d_Px_1_SG_D_3_25376) -> Px_1_SG_D_3/1
  w_SG_D_3/1 -> d_psi_d_SG_D_3_block/9(State_w_SG_D_3_932f2), d_psi_q_SG_D_3_block/9(State_w_SG_D_3_c59e4), d_V_f_SG_D_3_block/13(State_w_SG_D_3_3aaab), d_w_SG_D_3_block/1(State_w_SG_D_3_20cab), d_V_f_SG_D_3_block/8(State_w_SG_D_3_9905c), d_theta_SG_D_3_block/1(State_w_SG_D_3_5b30a), d_Px_1_SG_D_3_block/2(State_w_SG_D_3_a2340), d_T_m_SG_D_3_block/1(State_w_SG_D_3_a0204), d_Px_2_SG_D_3_block/4(State_w_SG_D_3_5fd48), w_SG_D_3_out_block/1(State_w_SG_D_3_85843), d_Px_3_SG_D_3_block/6(State_w_SG_D_3_1436e)
  d_T_m_SG_D_3_block/1(Blockout_d_T_m_SG_D_3_70e32) -> T_m_SG_D_3/1
  R_f_SG_D_3/1 -> d_V_f_SG_D_3_block/2(State_R_f_SG_D_3_59f10), d_R_f_SG_D_3_block/2(State_R_f_SG_D_3_30cf3)
  w_SG_D_3_out_block/1(Blockout_w_SG_D_3_out_7e4e6) -> w_SG_D_3_out/1
  d_Px_2_SG_D_3_block/1(Blockout_d_Px_2_SG_D_3_2a6eb) -> Px_2_SG_D_3/1
  d_w_SG_D_3_block/1(Blockout_d_w_SG_D_3_59b12) -> w_SG_D_3/1
  Px_1_SG_D_3/1 -> d_Px_1_SG_D_3_block/1(State_Px_1_SG_D_3_32a62), d_Px_3_SG_D_3_block/4(State_Px_1_SG_D_3_d42a9), d_Px_2_SG_D_3_block/2(State_Px_1_SG_D_3_a5179), d_Px_2_SG_D_3_block/3(State_Px_1_SG_D_3_97597), d_Px_3_SG_D_3_block/5(State_Px_1_SG_D_3_54980)
  d_theta_SG_D_3_block/1(Blockout_d_theta_SG_D_3_099ad) -> theta_SG_D_3/1
  d_Px_3_SG_D_3_block/1(Blockout_d_Px_3_SG_D_3_0e541) -> Px_3_SG_D_3/1
  T_m_SG_D_3/1 -> d_T_m_SG_D_3_block/2(State_T_m_SG_D_3_0a98b), d_w_SG_D_3_block/2(State_T_m_SG_D_3_017f4)
  psi_q_SG_D_3/1 -> d_psi_d_SG_D_3_block/8(State_psi_q_SG_D_3_cae6b), d_psi_q_SG_D_3_block/3(State_psi_q_SG_D_3_f40ab), d_psi_gq_SG_D_3_block/6(State_psi_q_SG_D_3_4df2f), d_psi_gq_SG_D_3_block/9(State_psi_q_SG_D_3_81891), d_psi_kq_SG_D_3_block/5(State_psi_q_SG_D_3_faf2a), d_V_f_SG_D_3_block/7(State_psi_q_SG_D_3_e11c8), i_d_SG_D_3_block/3(State_psi_q_SG_D_3_5bb1f), i_q_SG_D_3_block/3(State_psi_q_SG_D_3_c30f0), d_w_SG_D_3_block/7(State_psi_q_SG_D_3_58c30), T_e_SG_D_3_block/4(State_psi_q_SG_D_3_76dcc), d_w_SG_D_3_block/6(State_psi_q_SG_D_3_83586), T_e_SG_D_3_block/5(State_psi_q_SG_D_3_c10b9), d_V_f_SG_D_3_block/11(State_psi_q_SG_D_3_30298)
  psi_d_SG_D_3/1 -> d_psi_fd_SG_D_3_block/9(State_psi_d_SG_D_3_2871d), d_psi_fd_SG_D_3_block/6(State_psi_d_SG_D_3_13ba3), d_psi_d_SG_D_3_block/2(State_psi_d_SG_D_3_7cd0f), d_psi_q_SG_D_3_block/8(State_psi_d_SG_D_3_d979d), d_w_SG_D_3_block/3(State_psi_d_SG_D_3_957f3), d_V_f_SG_D_3_block/12(State_psi_d_SG_D_3_11840), i_q_SG_D_3_block/6(State_psi_d_SG_D_3_3005d), T_e_SG_D_3_block/1(State_psi_d_SG_D_3_1c144), T_e_SG_D_3_block/7(State_psi_d_SG_D_3_65d7f), d_V_f_SG_D_3_block/5(State_psi_d_SG_D_3_10634), d_psi_1d_SG_D_3_block/4(State_psi_d_SG_D_3_323ac), d_w_SG_D_3_block/9(State_psi_d_SG_D_3_c720b), i_d_SG_D_3_block/6(State_psi_d_SG_D_3_e794c)
  v_d_SG_D_3/1 -> d_psi_d_SG_D_3_block/4(Input_v_d_SG_D_3_5796f), d_psi_q_SG_D_3_block/4(Input_v_d_SG_D_3_58a7d)
  v_q_SG_D_3/1 -> d_psi_d_SG_D_3_block/6(Input_v_q_SG_D_3_9c4e0), d_psi_q_SG_D_3_block/6(Input_v_q_SG_D_3_adcaa)
  theta_SG_D_3/1 -> d_psi_q_SG_D_3_block/7(State_theta_SG_D_3_acab9), d_psi_q_SG_D_3_block/5(State_theta_SG_D_3_99845), d_psi_d_SG_D_3_block/5(State_theta_SG_D_3_13722), i_d_SG_D_3_block/4(State_theta_SG_D_3_64bc2), i_d_SG_D_3_block/8(State_theta_SG_D_3_abf6f), d_psi_d_SG_D_3_block/7(State_theta_SG_D_3_a9183), i_q_SG_D_3_block/4(State_theta_SG_D_3_b3699), i_q_SG_D_3_block/8(State_theta_SG_D_3_2de5d), theta_SG_D_3_out_block/1(State_theta_SG_D_3_d5a12)
  psi_gq_SG_D_3/1 -> d_psi_q_SG_D_3_block/1(State_psi_gq_SG_D_3_0e7f2), d_psi_gq_SG_D_3_block/2(State_psi_gq_SG_D_3_d037a), d_psi_gq_SG_D_3_block/4(State_psi_gq_SG_D_3_a5194), d_psi_gq_SG_D_3_block/7(State_psi_gq_SG_D_3_8a365), d_w_SG_D_3_block/4(State_psi_gq_SG_D_3_70980), d_psi_kq_SG_D_3_block/3(State_psi_gq_SG_D_3_e82df), d_psi_kq_SG_D_3_block/1(State_psi_gq_SG_D_3_080c6), d_V_f_SG_D_3_block/9(State_psi_gq_SG_D_3_2f4fc), i_d_SG_D_3_block/1(State_psi_gq_SG_D_3_b8fc9), T_e_SG_D_3_block/2(State_psi_gq_SG_D_3_42e3f), d_psi_gq_SG_D_3_block/1(State_psi_gq_SG_D_3_a5045), i_q_SG_D_3_block/1(State_psi_gq_SG_D_3_ba53f)
  d_psi_kq_SG_D_3_block/1(Blockout_d_psi_kq_SG_D_3_45068) -> psi_kq_SG_D_3/1
  psi_1d_SG_D_3/1 -> d_psi_fd_SG_D_3_block/3(State_psi_1d_SG_D_3_2594f), d_psi_fd_SG_D_3_block/5(State_psi_1d_SG_D_3_6227c), d_psi_fd_SG_D_3_block/8(State_psi_1d_SG_D_3_d606f), d_psi_d_SG_D_3_block/1(State_psi_1d_SG_D_3_011cf), d_psi_1d_SG_D_3_block/1(State_psi_1d_SG_D_3_a0749), d_psi_1d_SG_D_3_block/3(State_psi_1d_SG_D_3_a47c4), d_w_SG_D_3_block/8(State_psi_1d_SG_D_3_95783), i_d_SG_D_3_block/5(State_psi_1d_SG_D_3_c5249), d_V_f_SG_D_3_block/4(State_psi_1d_SG_D_3_55945), i_q_SG_D_3_block/5(State_psi_1d_SG_D_3_87d21), T_e_SG_D_3_block/6(State_psi_1d_SG_D_3_ba052)
  psi_kq_SG_D_3/1 -> d_psi_q_SG_D_3_block/2(State_psi_kq_SG_D_3_f91e2), d_psi_gq_SG_D_3_block/3(State_psi_kq_SG_D_3_553f5), d_psi_gq_SG_D_3_block/5(State_psi_kq_SG_D_3_b8f3d), d_psi_kq_SG_D_3_block/2(State_psi_kq_SG_D_3_95f78), d_psi_kq_SG_D_3_block/4(State_psi_kq_SG_D_3_7c5b6), d_psi_gq_SG_D_3_block/8(State_psi_kq_SG_D_3_f4b71), d_V_f_SG_D_3_block/10(State_psi_kq_SG_D_3_7553e), i_q_SG_D_3_block/2(State_psi_kq_SG_D_3_ac7b7), T_e_SG_D_3_block/3(State_psi_kq_SG_D_3_2048a), i_d_SG_D_3_block/2(State_psi_kq_SG_D_3_ab859), d_w_SG_D_3_block/5(State_psi_kq_SG_D_3_c1afd)
  Px_2_SG_D_3/1 -> d_Px_2_SG_D_3_block/1(State_Px_2_SG_D_3_1f8e6), d_Px_3_SG_D_3_block/3(State_Px_2_SG_D_3_1a96a), d_Px_3_SG_D_3_block/2(State_Px_2_SG_D_3_e9479)
  psi_fd_SG_D_3/1 -> d_psi_fd_SG_D_3_block/2(State_psi_fd_SG_D_3_56bbf), d_psi_fd_SG_D_3_block/4(State_psi_fd_SG_D_3_2cf4f), d_psi_d_SG_D_3_block/3(State_psi_fd_SG_D_3_3b99c), d_psi_1d_SG_D_3_block/2(State_psi_fd_SG_D_3_90ea7), d_psi_fd_SG_D_3_block/7(State_psi_fd_SG_D_3_0f1b2), i_d_SG_D_3_block/7(State_psi_fd_SG_D_3_7ea81), d_V_f_SG_D_3_block/6(State_psi_fd_SG_D_3_56622), d_psi_1d_SG_D_3_block/5(State_psi_fd_SG_D_3_e5548), d_w_SG_D_3_block/10(State_psi_fd_SG_D_3_55350), d_psi_fd_SG_D_3_block/10(State_psi_fd_SG_D_3_ef464), i_q_SG_D_3_block/7(State_psi_fd_SG_D_3_35851), T_e_SG_D_3_block/8(State_psi_fd_SG_D_3_c97e9)
  d_V_f_SG_D_3_block/1(Blockout_d_V_f_SG_D_3_23441) -> V_f_SG_D_3/1
  theta_SG_D_3_out_block/1(Blockout_theta_SG_D_3_out_f4538) -> theta_SG_D_3_out/1
  i_d_SG_D_3_block/1(Blockout_i_d_SG_D_3_ca1dd) -> i_d_SG_D_3/1
  d_psi_d_SG_D_3_block/1(Blockout_d_psi_d_SG_D_3_79ce6) -> psi_d_SG_D_3/1
  d_R_f_SG_D_3_block/1(Blockout_d_R_f_SG_D_3_c0cf4) -> R_f_SG_D_3/1
  d_psi_q_SG_D_3_block/1(Blockout_d_psi_q_SG_D_3_0df16) -> psi_q_SG_D_3/1
  i_q_SG_D_3_block/1(Blockout_i_q_SG_D_3_68df7) -> i_q_SG_D_3/1
  d_psi_gq_SG_D_3_block/1(Blockout_d_psi_gq_SG_D_3_637a0) -> psi_gq_SG_D_3/1
  T_e_SG_D_3_block/1(Blockout_T_e_SG_D_3_1d3ff) -> T_e_SG_D_3/1
  d_psi_1d_SG_D_3_block/1(Blockout_d_psi_1d_SG_D_3_d513f) -> psi_1d_SG_D_3/1
  V_f_SG_D_3/1 -> d_E_fd_SG_D_3_block/2(State_V_f_SG_D_3_40669), d_V_f_SG_D_3_block/14(State_V_f_SG_D_3_b14e2)
  Px_3_SG_D_3/1 -> d_Px_3_SG_D_3_block/1(State_Px_3_SG_D_3_77d5b), d_V_f_SG_D_3_block/3(State_Px_3_SG_D_3_92418)
  d_E_fd_SG_D_3_block/1(Blockout_d_E_fd_SG_D_3_8845a) -> E_fd_SG_D_3/1
  E_fd_SG_D_3/1 -> d_V_f_SG_D_3_block/1(State_E_fd_SG_D_3_5c701), d_E_fd_SG_D_3_block/1(State_E_fd_SG_D_3_7cd07), d_R_f_SG_D_3_block/1(State_E_fd_SG_D_3_c60c1), d_psi_fd_SG_D_3_block/1(State_E_fd_SG_D_3_08aad)
  d_psi_fd_SG_D_3_block/1(Blockout_d_psi_fd_SG_D_3_6ae4a) -> psi_fd_SG_D_3/1

== system case3/AC_1/d_id_line_1_4_block ==
  note: d_id_line_1_4 in case3
      | $376.991118430775\,\mathrm{iq}_{\mathrm{line},1,4}+6255.26744708076\,\mathrm{vd}_{\mathrm{bus},1}-6255.26744708076\,\mathrm{vd}_{\mathrm{bus},4}$
      | Automatically generated on 2025-10-31 19:02:15 .
  State_iq_line_1_4_fc81e : Inport
  State_vd_bus_1_32af8 : Inport  Port=2
  State_vd_bus_4_baee6 : Inport  Port=3
  Add_c259a : Sum
  Constant_376.991118430775_feae6 : Constant  Value=376.991118430775
  Constant_6255.26744708076_007a8 : Constant  Value=6255.26744708076
  Constant_6255.26744708076_c140a : Constant  Value=6255.26744708076
  Product_00639 : Product
  Product_61903 : Product
  Product_ee6da : Product
  Subtract_0aa7d : Sum  Inputs=+-
  Blockout_d_id_line_1_4_f5e01 : Outport
  wires:
  Constant_376.991118430775_feae6/1 -> Product_00639/1
  Product_ee6da/1 -> Add_c259a/2
  State_iq_line_1_4_fc81e/1 -> Product_00639/2
  Subtract_0aa7d/1 -> Blockout_d_id_line_1_4_f5e01/1
  Constant_6255.26744708076_c140a/1 -> Product_ee6da/1
  Product_00639/1 -> Add_c259a/1
  State_vd_bus_1_32af8/1 -> Product_ee6da/2
  Constant_6255.26744708076_007a8/1 -> Product_61903/1
  State_vd_bus_4_baee6/1 -> Product_61903/2
  Add_c259a/1 -> Subtract_0aa7d/1
  Product_61903/1 -> Subtract_0aa7d/2

== system case3/AC_1/d_id_line_3_6_block ==
  note: d_id_line_3_6 in case3
      | $376.991118430775\,\mathrm{iq}_{\mathrm{line},3,6}+6148.52226880293\,\mathrm{vd}_{\mathrm{bus},3}-6148.52226880293\,\mathrm{vd}_{\mathrm{bus},6}$
      | Automatically generated on 2025-10-31 19:02:22 .
  State_iq_line_3_6_ad0cd : Inport
  State_vd_bus_3_f9f03 : Inport  Port=2
  State_vd_bus_6_86153 : Inport  Port=3
  Add_0d2da : Sum
  Constant_376.991118430775_45c7c : Constant  Value=376.991118430775
  Constant_6148.52226880293_0c897 : Constant  Value=6148.52226880293
  Constant_6148.52226880293_e2bb8 : Constant  Value=6148.52226880293
  Product_37b3d : Product
  Product_5d303 : Product
  Product_a6fe7 : Product
  Subtract_722bf : Sum  Inputs=+-
  Blockout_d_id_line_3_6_3490b : Outport
  wires:
  State_vd_bus_3_f9f03/1 -> Product_a6fe7/2
  Constant_376.991118430775_45c7c/1 -> Product_5d303/1
  Product_a6fe7/1 -> Add_0d2da/2
  State_iq_line_3_6_ad0cd/1 -> Product_5d303/2
  Constant_6148.52226880293_0c897/1 -> Product_a6fe7/1
  Product_5d303/1 -> Add_0d2da/1
  Constant_6148.52226880293_e2bb8/1 -> Product_37b3d/1
  State_vd_bus_6_86153/1 -> Product_37b3d/2
  Add_0d2da/1 -> Subtract_722bf/1
  Product_37b3d/1 -> Subtract_722bf/2
  Subtract_722bf/1 -> Blockout_d_id_line_3_6_3490b/1

== system case3/AC_1/d_id_line_4_5_block ==
  note: d_id_line_4_5 in case3
      | $376.991118430775\,\mathrm{iq}_{\mathrm{line},4,5}-71.2470020354664\,\mathrm{id}_{\mathrm{line},4,5}+3916.3413581723\,\mathrm{vd}_{\mathrm{bus},4}-3916.3413581723\,\mathrm{vd}_{\mathrm{bus},5}$
      | Automatically generated on 2025-10-31 19:02:17 .
  State_id_line_4_5_125e0 : Inport
  State_iq_line_4_5_cfaf0 : Inport  Port=2
  State_vd_bus_4_48529 : Inport  Port=3
  State_vd_bus_5_31906 : Inport  Port=4
  Add_22fb2 : Sum
  Add_73a82 : Sum
  Constant_-71.2470020354664_15ba9 : Constant  Value=-71.2470020354664
  Constant_376.991118430775_eb3ea : Constant  Value=376.991118430775
  Constant_3916.3413581723_01c94 : Constant  Value=3916.3413581723
  Constant_3916.3413581723_3450e : Constant  Value=3916.3413581723
  Product_84f3a : Product
  Product_88a75 : Product
  Product_c1515 : Product
  Product_f828b : Product
  Subtract_510c0 : Sum  Inputs=+-
  Blockout_d_id_line_4_5_12103 : Outport
  wires:
  Constant_-71.2470020354664_15ba9/1 -> Product_84f3a/1
  Product_88a75/1 -> Add_73a82/2
  State_id_line_4_5_125e0/1 -> Product_84f3a/2
  Constant_376.991118430775_eb3ea/1 -> Product_88a75/1
  State_iq_line_4_5_cfaf0/1 -> Product_88a75/2
  Product_84f3a/1 -> Add_73a82/1
  Constant_3916.3413581723_01c94/1 -> Product_c1515/1
  State_vd_bus_4_48529/1 -> Product_c1515/2
  Add_73a82/1 -> Add_22fb2/1
  Product_c1515/1 -> Add_22fb2/2
  Constant_3916.3413581723_3450e/1 -> Product_f828b/1
  State_vd_bus_5_31906/1 -> Product_f828b/2
  Add_22fb2/1 -> Subtract_510c0/1
  Product_f828b/1 -> Subtract_510c0/2
  Subtract_510c0/1 -> Blockout_d_id_line_4_5_12103/1

== system case3/AC_1/d_id_line_5_6_block ==
  note: d_id_line_5_6 in case3
      | $376.991118430775\,\mathrm{iq}_{\mathrm{line},5,6}-88.4547554682538\,\mathrm{id}_{\mathrm{line},5,6}+2119.43179383442\,\mathrm{vd}_{\mathrm{bus},5}-2119.43179383442\,\mathrm{vd}_{\mathrm{bus},6}$
      | Automatically generated on 2025-10-31 19:02:19 .
  State_id_line_5_6_11d83 : Inport
  State_iq_line_5_6_14e07 : Inport  Port=2
  State_vd_bus_5_794d2 : Inport  Port=3
  State_vd_bus_6_02860 : Inport  Port=4
  Add_b01e4 : Sum
  Add_eb684 : Sum
  Constant_-88.4547554682538_c11b1 : Constant  Value=-88.4547554682538
  Constant_2119.43179383442_2c394 : Constant  Value=2119.43179383442
  Constant_2119.43179383442_ee9b3 : Constant  Value=2119.43179383442
  Constant_376.991118430775_6ba81 : Constant  Value=376.991118430775
  Product_4a736 : Product
  Product_4b7e3 : Product
  Product_bea95 : Product
  Product_e48b9 : Product
  Subtract_b0a4a : Sum  Inputs=+-
  Blockout_d_id_line_5_6_8629c : Outport
  wires:
  Constant_-88.4547554682538_c11b1/1 -> Product_4b7e3/1
  Product_e48b9/1 -> Add_eb684/2
  State_id_line_5_6_11d83/1 -> Product_4b7e3/2
  Constant_376.991118430775_6ba81/1 -> Product_e48b9/1
  Product_4b7e3/1 -> Add_eb684/1
  State_iq_line_5_6_14e07/1 -> Product_e48b9/2
  Constant_2119.43179383442_ee9b3/1 -> Product_4a736/1
  Product_bea95/1 -> Subtract_b0a4a/2
  State_vd_bus_5_794d2/1 -> Product_4a736/2
  Add_eb684/1 -> Add_b01e4/1
  Product_4a736/1 -> Add_b01e4/2
  Constant_2119.43179383442_2c394/1 -> Product_bea95/1
  State_vd_bus_6_02860/1 -> Product_bea95/2
  Add_b01e4/1 -> Subtract_b0a4a/1
  Subtract_b0a4a/1 -> Blockout_d_id_line_5_6_8629c/1

== system case3/AC_1/d_id_line_6_7_block ==
  note: d_id_line_6_7 in case3
      | $376.991118430775\,\mathrm{iq}_{\mathrm{line},6,7}-45.5189179671035\,\mathrm{id}_{\mathrm{line},6,7}+3574.43854118901\,\mathrm{vd}_{\mathrm{bus},6}-3574.43854118901\,\mathrm{vd}_{\mathrm{bus},7}$
      | Automatically generated on 2025-10-31 19:02:24 .
  State_id_line_6_7_3cec9 : Inport
  State_iq_line_6_7_7db22 : Inport  Port=2
  State_vd_bus_6_9819c : Inport  Port=3
  State_vd_bus_7_1ec6b : Inport  Port=4
  Add_dc226 : Sum
  Add_de6c4 : Sum
  Constant_-45.5189179671035_a890b : Constant  Value=-45.5189179671035
  Constant_3574.43854118901_08f95 : Constant  Value=3574.43854118901
  Constant_3574.43854118901_2fa2e : Constant  Value=3574.43854118901
  Constant_376.991118430775_6975d : Constant  Value=376.991118430775
  Product_355e9 : Product
  Product_44219 : Product
  Product_a363a : Product
  Product_c4ae5 : Product
  Subtract_6a589 : Sum  Inputs=+-
  Blockout_d_id_line_6_7_d9830 : Outport
  wires:
  Constant_-45.5189179671035_a890b/1 -> Product_44219/1
  Product_a363a/1 -> Add_de6c4/2
  State_id_line_6_7_3cec9/1 -> Product_44219/2
  Constant_376.991118430775_6975d/1 -> Product_a363a/1
  State_iq_line_6_7_7db22/1 -> Product_a363a/2
  Product_44219/1 -> Add_de6c4/1
  Constant_3574.43854118901_2fa2e/1 -> Product_355e9/1
  State_vd_bus_6_9819c/1 -> Product_355e9/2
  Add_de6c4/1 -> Add_dc226/1
  Product_355e9/1 -> Add_dc226/2
  Constant_3574.43854118901_08f95/1 -> Product_c4ae5/1
  State_vd_bus_7_1ec6b/1 -> Product_c4ae5/2
  Add_dc226/1 -> Subtract_6a589/1
  Product_c4ae5/1 -> Subtract_6a589/2
  Subtract_6a589/1 -> Blockout_d_id_line_6_7_d9830/1

== system case3/AC_1/d_id_line_7_8_block ==
  note: d_id_line_7_8 in case3
      | $376.991118430775\,\mathrm{iq}_{\mathrm{line},7,8}-45.5189179671035\,\mathrm{id}_{\mathrm{line},7,8}+5004.21395766461\,\mathrm{vd}_{\mathrm{bus},7}-5004.21395766461\,\mathrm{vd}_{\mathrm{bus},8}$
      | Automatically generated on 2025-10-31 19:02:27 .
  State_id_line_7_8_104c2 : Inport
  State_iq_line_7_8_8ab2b : Inport  Port=2
  State_vd_bus_7_bda80 : Inport  Port=3
  State_vd_bus_8_b8c1f : Inport  Port=4
  Add_c512f : Sum
  Add_e0116 : Sum
  Constant_-45.5189179671035_d8557 : Constant  Value=-45.5189179671035
  Constant_376.991118430775_435ed : Constant  Value=376.991118430775
  Constant_5004.21395766461_ccfb2 : Constant  Value=5004.21395766461
  Constant_5004.21395766461_e544c : Constant  Value=5004.21395766461
  Product_04ab6 : Product
  Product_264a2 : Product
  Product_ae394 : Product
  Product_de465 : Product
  Subtract_8efb8 : Sum  Inputs=+-
  Blockout_d_id_line_7_8_1308e : Outport
  wires:
  Constant_-45.5189179671035_d8557/1 -> Product_264a2/1
  Product_ae394/1 -> Add_e0116/2
  State_id_line_7_8_104c2/1 -> Product_264a2/2
  Constant_376.991118430775_435ed/1 -> Product_ae394/1
  Product_264a2/1 -> Add_e0116/1
  State_iq_line_7_8_8ab2b/1 -> Product_ae394/2
  Constant_5004.21395766461_e544c/1 -> Product_de465/1
  State_vd_bus_7_bda80/1 -> Product_de465/2
  Add_e0116/1 -> Add_c512f/1
  Product_de465/1 -> Add_c512f/2
  Constant_5004.21395766461_ccfb2/1 -> Product_04ab6/1
  State_vd_bus_8_b8c1f/1 -> Product_04ab6/2
  Add_c512f/1 -> Subtract_8efb8/1
  Product_04ab6/1 -> Subtract_8efb8/2
  Subtract_8efb8/1 -> Blockout_d_id_line_7_8_1308e/1

== system case3/AC_1/d_id_line_8_2_block ==
  note: d_id_line_8_2 in case3
      | $376.991118430775\,\mathrm{iq}_{\mathrm{line},8,2}-5764.85447922963\,\mathrm{vd}_{\mathrm{bus},2}+5764.85447922963\,\mathrm{vd}_{\mathrm{bus},8}$
      | Automatically generated on 2025-10-31 19:02:30 .
  State_iq_line_8_2_c2450 : Inport
  State_vd_bus_2_982da : Inport  Port=2
  State_vd_bus_8_1a12f : Inport  Port=3
  Add_12471 : Sum
  Constant_376.991118430775_b5bdc : Constant  Value=376.991118430775
  Constant_5764.85447922963_bb01d : Constant  Value=5764.85447922963
  Constant_5764.85447922963_efb12 : Constant  Value=5764.85447922963
  Product_32540 : Product
  Product_951ef : Product
  Product_ce2ea : Product
  Subtract_0dc90 : Sum  Inputs=+-
  Blockout_d_id_line_8_2_922a4 : Outport
  wires:
  State_vd_bus_2_982da/1 -> Product_32540/2
  Constant_376.991118430775_b5bdc/1 -> Product_ce2ea/1
  Product_32540/1 -> Subtract_0dc90/2
  State_iq_line_8_2_c2450/1 -> Product_ce2ea/2
  Constant_5764.85447922963_bb01d/1 -> Product_32540/1
  Product_ce2ea/1 -> Subtract_0dc90/1
  Constant_5764.85447922963_efb12/1 -> Product_951ef/1
  State_vd_bus_8_1a12f/1 -> Product_951ef/2
  Subtract_0dc90/1 -> Add_12471/1
  Product_951ef/1 -> Add_12471/2
  Add_12471/1 -> Blockout_d_id_line_8_2_922a4/1

== system case3/AC_1/d_id_line_8_9_block ==
  note: d_id_line_8_9 in case3
      | $376.991118430775\,\mathrm{iq}_{\mathrm{line},8,9}-76.6354307608378\,\mathrm{id}_{\mathrm{line},8,9}+2237.90934752703\,\mathrm{vd}_{\mathrm{bus},8}-2237.90934752703\,\mathrm{vd}_{\mathrm{bus},9}$
      | Automatically generated on 2025-10-31 19:02:32 .
  State_id_line_8_9_8f4c6 : Inport
  State_iq_line_8_9_f80cf : Inport  Port=2
  State_vd_bus_8_789f7 : Inport  Port=3
  State_vd_bus_9_a0458 : Inport  Port=4
  Add_16278 : Sum
  Add_9c183 : Sum
  Constant_-76.6354307608378_6ecb3 : Constant  Value=-76.6354307608378
  Constant_2237.90934752703_a32a9 : Constant  Value=2237.90934752703
  Constant_2237.90934752703_fa9ec : Constant  Value=2237.90934752703
  Constant_376.991118430775_2734d : Constant  Value=376.991118430775
  Product_3c020 : Product
  Product_bbd1a : Product
  Product_d57e7 : Product
  Product_dbffb : Product
  Subtract_77401 : Sum  Inputs=+-
  Blockout_d_id_line_8_9_9c30d : Outport
  wires:
  Constant_-76.6354307608378_6ecb3/1 -> Product_bbd1a/1
  Product_dbffb/1 -> Add_9c183/2
  State_id_line_8_9_8f4c6/1 -> Product_bbd1a/2
  Constant_376.991118430775_2734d/1 -> Product_dbffb/1
  State_iq_line_8_9_f80cf/1 -> Product_dbffb/2
  Product_bbd1a/1 -> Add_9c183/1
  Constant_2237.90934752703_fa9ec/1 -> Product_d57e7/1
  State_vd_bus_8_789f7/1 -> Product_d57e7/2
  Add_9c183/1 -> Add_16278/1
  Product_d57e7/1 -> Add_16278/2
  Constant_2237.90934752703_a32a9/1 -> Product_3c020/1
  State_vd_bus_9_a0458/1 -> Product_3c020/2
  Add_16278/1 -> Subtract_77401/1
  Product_3c020/1 -> Subtract_77401/2
  Subtract_77401/1 -> Blockout_d_id_line_8_9_9c30d/1

== system case3/AC_1/d_id_line_9_4_block ==
  note: d_id_line_9_4 in case3
      | $376.991118430775\,\mathrm{iq}_{\mathrm{line},9,4}-45.3614130606429\,\mathrm{id}_{\mathrm{line},9,4}-4238.86358766884\,\mathrm{vd}_{\mathrm{bus},4}+4238.86358766884\,\mathrm{vd}_{\mathrm{bus},9}$
      | Automatically generated on 2025-10-31 19:02:35 .
  State_id_line_9_4_02a1a : Inport
  State_iq_line_9_4_819ce : Inport  Port=2
  State_vd_bus_4_32929 : Inport  Port=3
  State_vd_bus_9_a7a68 : Inport  Port=4
  Add_095b6 : Sum
  Add_b75a8 : Sum
  Constant_-45.3614130606429_7678d : Constant  Value=-45.3614130606429
  Constant_376.991118430775_8f303 : Constant  Value=376.991118430775
  Constant_4238.86358766884_01688 : Constant  Value=4238.86358766884
  Constant_4238.86358766884_7ab79 : Constant  Value=4238.86358766884
  Product_1c3f4 : Product
  Product_8b027 : Product
  Product_d0d75 : Product
  Product_d290f : Product
  Subtract_d20a0 : Sum  Inputs=+-
  Blockout_d_id_line_9_4_f8e36 : Outport
  wires:
  Constant_-45.3614130606429_7678d/1 -> Product_8b027/1
  Product_1c3f4/1 -> Add_095b6/2
  State_id_line_9_4_02a1a/1 -> Product_8b027/2
  Constant_376.991118430775_8f303/1 -> Product_1c3f4/1
  Product_8b027/1 -> Add_095b6/1
  State_iq_line_9_4_819ce/1 -> Product_1c3f4/2
  Constant_4238.86358766884_01688/1 -> Product_d290f/1
  State_vd_bus_4_32929/1 -> Product_d290f/2
  Add_095b6/1 -> Subtract_d20a0/1
  Product_d290f/1 -> Subtract_d20a0/2
  Constant_4238.86358766884_7ab79/1 -> Product_d0d75/1
  Subtract_d20a0/1 -> Add_b75a8/1
  State_vd_bus_9_a7a68/1 -> Product_d0d75/2
  Product_d0d75/1 -> Add_b75a8/2
  Add_b75a8/1 -> Blockout_d_id_line_9_4_f8e36/1

== system case3/AC_1/d_id_load_5_block ==
  note: d_id_load_5 in case3
      | $376.991118430775\,\mathrm{iq}_{\mathrm{load},5}-1229.33491779484\,\mathrm{id}_{\mathrm{load},5}+1333.35238164348\,\mathrm{vd}_{\mathrm{bus},5}$
      | Automatically generated on 2025-10-31 19:02:08 .
  State_id_load_5_21183 : Inport
  State_iq_load_5_e6e38 : Inport  Port=2
  State_vd_bus_5_9c3f5 : Inport  Port=3
  Add_033c6 : Sum
  Add_756da : Sum
  Constant_-1229.33491779484_79908 : Constant  Value=-1229.33491779484
  Constant_1333.35238164348_81c03 : Constant  Value=1333.35238164348
  Constant_376.991118430775_3d957 : Constant  Value=376.991118430775
  Product_67fc3 : Product
  Product_afb5e : Product
  Product_b3f48 : Product
  Blockout_d_id_load_5_20828 : Outport
  wires:
  Constant_-1229.33491779484_79908/1 -> Product_afb5e/1
  Product_67fc3/1 -> Add_033c6/2
  State_id_load_5_21183/1 -> Product_afb5e/2
  Constant_376.991118430775_3d957/1 -> Product_67fc3/1
  Product_b3f48/1 -> Add_756da/2
  State_iq_load_5_e6e38/1 -> Product_67fc3/2
  Product_afb5e/1 -> Add_033c6/1
  Constant_1333.35238164348_81c03/1 -> Product_b3f48/1
  State_vd_bus_5_9c3f5/1 -> Product_b3f48/2
  Add_033c6/1 -> Add_756da/1
  Add_756da/1 -> Blockout_d_id_load_5_20828/1
